simulink model "IdealTrackGenerator"  (R2017a)
settings: Solver=ode4  StartTime=0.0  StopTime=Tend  FixedStep=Ts  RelTol=1e-3  EnableMultiTasking=on
values from neighbouring files (symbols this model uses):
  k_overshoot = 8    [IdealTrack_v3_longlat.m]
  TDs = 20    [IdealTrack_v3_longlat.m]
  Ttry = TDe - TDs    (= 10)    [IdealTrack_v3_longlat.m]
  x_tempt = x_tempt + 0.01*e_x    [IdealTrack_v3_longlat.m]
  y_tempt = y_tempt + 0.05*e_y    [IdealTrack_v3_longlat.m]
  z_tempt = z_tempt + 0.05*e_z    [IdealTrack_v3_longlat.m]
settings Model: Creator=WhisPer  LastModifiedBy=ttjr11
settings DataIOCC: LimitDataPoints=on  SaveFormat=Array
settings OptimizationCC: LifeSpan=inf
settings DebuggingCC: UnderspecifiedInitializationDetection=Classic  MergeDetectMultiDrivingBlocksExec=none  SolverPrmCheckMsg=warning  AllowSymbolicDim=off  StateNameClashWarn=warning  SFUnexpectedBacktrackingDiag=warning  SFNoUnconditionalDefaultTransitionDiag=warning  SFExecutionAtInitializationDiag=none
settings HardwareCC: ProdBitPerPointer=32  ProdBitPerSizeT=32  ProdBitPerPtrDiffT=32  ProdLargestAtomicFloat=None  ProdIntDivRoundTo=Undefined  ProdEndianess=Unspecified  ProdWordSize=32  ProdHWDeviceType=32-bit Generic
settings ModelReferenceCC: PropagateSignalLabelsOutOfModel=off
settings GRTTargetCC: TargetLangStandard=C89/C90 (ANSI)  GeneratePreprocessorConditionals=Disable all
settings ConfigComp: CovMetricSettings=dw  CovHtmlReporting=on  CovSaveCumulativeToWorkspaceVar=on  CovSaveSingleToWorkspaceVar=on  CovExternalEMLEnable=off

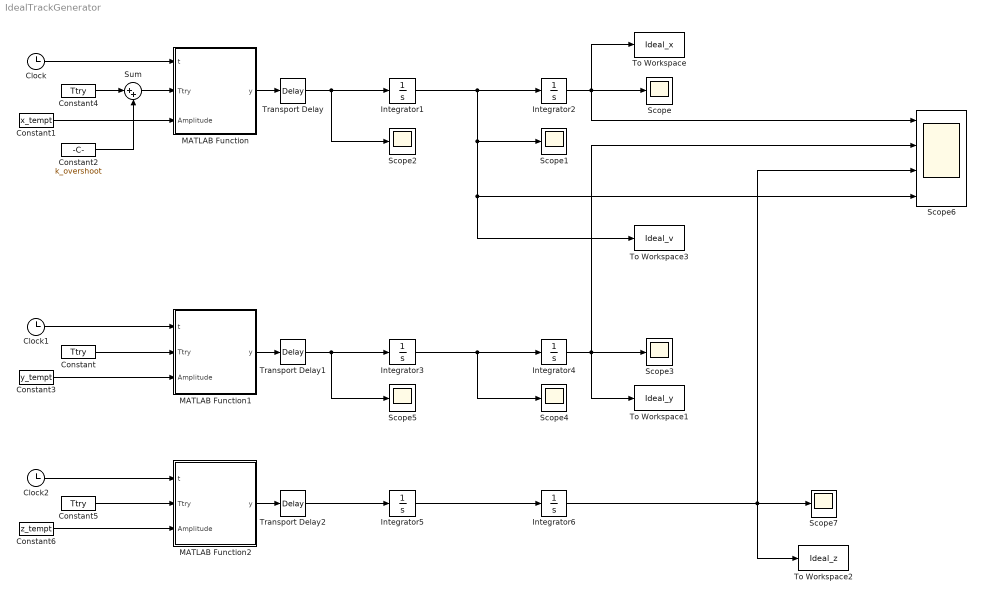
== system IdealTrackGenerator ==
  Clock : Clock
  Clock1 : Clock
  Clock2 : Clock
  Constant : Constant  Value=Ttry
  Constant1 : Constant  Value=x_tempt
  Constant2 : Constant  Value=k_overshoot
  Constant3 : Constant  Value=y_tempt
  Constant4 : Constant  Value=Ttry
  Constant5 : Constant  Value=Ttry
  Constant6 : Constant  Value=z_tempt
  Integrator{1..6} (6 alike) : Integrator
  MATLAB Function : MATLAB Function  TreatAsAtomicUnit=on
  MATLAB Function1 : MATLAB Function  TreatAsAtomicUnit=on
  MATLAB Function2 : MATLAB Function  TreatAsAtomicUnit=on
  Scope{,1..5,7} (7 alike) : Scope
  Scope6 : Scope  NumInputPorts=4
  Sum : Sum  Inputs=|++
  To Workspace : ToWorkspace  VariableName=Ideal_x  SampleTime=-1
  To Workspace1 : ToWorkspace  VariableName=Ideal_y  SampleTime=-1
  To Workspace2 : ToWorkspace  VariableName=Ideal_z  SampleTime=-1
  To Workspace3 : ToWorkspace  VariableName=Ideal_v  SampleTime=-1
  Transport Delay : TransportDelay  DelayTime=TDs
  Transport Delay1 : TransportDelay  DelayTime=TDs
  Transport Delay2 : TransportDelay  DelayTime=TDs
  wires:
  Clock/1 -> MATLAB Function/1(t)
  Constant1/1 -> MATLAB Function/3(Amplitude)
  MATLAB Function/1(y) -> Transport Delay/1
  Integrator1/1 -> To Workspace3/1, Scope6/4, Scope1/1, Integrator2/1
  Integrator2/1 -> To Workspace/1, Scope/1, Scope6/1
  Clock1/1 -> MATLAB Function1/1(t)
  Constant3/1 -> MATLAB Function1/3(Amplitude)
  MATLAB Function1/1(y) -> Transport Delay1/1
  Integrator3/1 -> Scope4/1, Integrator4/1
  Integrator4/1 -> To Workspace1/1, Scope6/2, Scope3/1
  Constant/1 -> MATLAB Function1/2(Ttry)
  Constant4/1 -> Sum/1
  Sum/1 -> MATLAB Function/2(Ttry)
  Transport Delay/1 -> Scope2/1, Integrator1/1
  Transport Delay1/1 -> Scope5/1, Integrator3/1
  Constant2/1 -> Sum/2
  Clock2/1 -> MATLAB Function2/1(t)
  Constant6/1 -> MATLAB Function2/3(Amplitude)
  MATLAB Function2/1(y) -> Transport Delay2/1
  Constant5/1 -> MATLAB Function2/2(Ttry)
  Transport Delay2/1 -> Integrator5/1
  Integrator5/1 -> Integrator6/1
  Integrator6/1 -> To Workspace2/1, Scope6/3, Scope7/1

== matlab function IdealTrackGenerator/MATLAB Function1 ==
  data: t input; y output; Ttry input; Amplitude input
function y = fcn(t,Ttry,Amplitude)
% 加速度的形式：
% 在正方向上升，在rate*0.5*Ttry处下降，直到0.5*Ttry为0
% 然后在负方向下降，在(1-rate*0.5)*Ttry处上升，直到Ttry保持0不变
rate = 0.3; 
k1 = Amplitude/(rate*0.5*Ttry);
k2 = - Amplitude/((1-rate)*0.5*Ttry);
if t <= rate*0.5*Ttry
    y = k1*t;
elseif t <= (1-rate*0.5)*Ttry
    y = k2*t - 0.5*k2*Ttry;
elseif t <= Ttry
    y = k1*t - k1*Ttry;
else
    y = 0;
end

== matlab function IdealTrackGenerator/MATLAB Function ==
  data: t input; y output; Ttry input; Amplitude input
function y = fcn(t,Ttry,Amplitude)
% 加速度的形式：
% 在正方向上升，在rate*0.5*Ttry处下降，直到0.5*Ttry为0
% 然后在负方向下降，在(1-rate*0.5)*Ttry处上升，直到Ttry保持0不变
rate = 0.7; 
k1 = Amplitude/(rate*0.5*Ttry);
k2 = - Amplitude/((1-rate)*0.5*Ttry);
if t <= rate*0.5*Ttry
    y = k1*t;
elseif t <= (1-rate*0.5)*Ttry
    y = k2*t - 0.5*k2*Ttry;
elseif t <= Ttry
    y = k1*t - k1*Ttry;
else
    y = 0;
end

== matlab function IdealTrackGenerator/MATLAB Function2 ==
  data: t input; y output; Ttry input; Amplitude input
function y = fcn(t,Ttry,Amplitude)
% 加速度的形式：
% 在正方向上升，在rate*0.5*Ttry处下降，直到0.5*Ttry为0
% 然后在负方向下降，在(1-rate*0.5)*Ttry处上升，直到Ttry保持0不变
rate = 0.3; 
k1 = Amplitude/(rate*0.5*Ttry);
k2 = - Amplitude/((1-rate)*0.5*Ttry);
if t <= rate*0.5*Ttry
    y = k1*t;
elseif t <= (1-rate*0.5)*Ttry
    y = k2*t - 0.5*k2*Ttry;
elseif t <= Ttry
    y = k1*t - k1*Ttry;
else
    y = 0;
end
